simulink model "SigSourceBaseSignal"  (R2022b)
settings: Solver=VariableStepAuto  StartTime=0.0  StopTime=10.0  RelTol=1e-3
undefined symbols (not defined in the file): CarrierTs, CodeTs, gcbh, mdel, ModelInitial, rcfiltgaincompat, rsgenpoly, SignalSourceTs
libraries: commsynccomp2 x3, commblkintrlv2 x2, dspobslib x1, commblkcod2 x1, commfilt2 x1, commrandsrc3 x1, commdigbbndam3 x1, simulink x1, commdigbbndfm2 x1, commseqgen3 x1
settings Model: Creator=79327  LastModifiedBy=79327

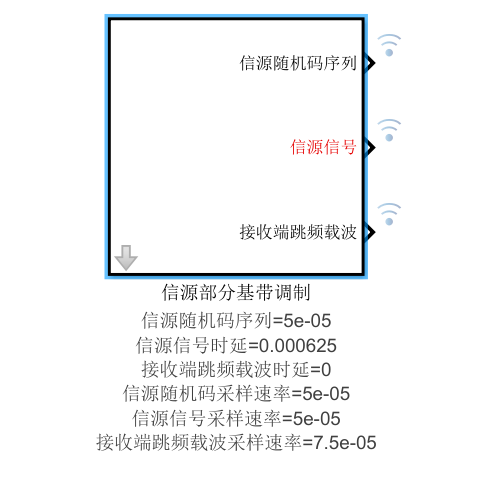
[thumbnail: Simulink's stored preview of the top-level diagram]
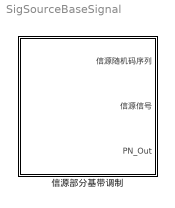
== system SigSourceBaseSignal ==
  信源部分基带调制 : Subsystem  InitFcn=ModelInitial(mdel,'信源部分基带调制',CodeTs,CarrierTs,SignalSourceTs)  TreatAsAtomicUnit=on  mask{SignalSource_Ts=SignalSourceTs, SampleFrame=3, M=15, PN_Generate=[1 0 0 0  0 1 1], PN_Init=[1 0 1 1 0 1], M_Freq=16, HopFrequencyStep=1e6, N=1500, Delay_HopFreq=0, Delay_SourceRand=5e-05, Delay_SignalSource=0.000625, CodeTs=CodeTs, CarrierTs=CarrierTs, SignalSourceTs=SignalSourceTs, T_HopFreq=7.5e-05, T_SourceRand=5e-05, T_SignalSource=5e-05}
      mask prompts: SignalSource_Ts "信源采样时间"; SampleFrame "信源随机码每帧的采样数"; M "信源M进制"; PN_Generate "PN生成器序列"; PN_Init "PN初始状态"; M_Freq "跳频的M进制"; HopFrequencyStep "跳频间隔"; N "输出跳频载波信号的维度"; Delay_HopFreq "接收端跳频载波的时延"; Delay_SourceRand "信源随机码的时延"; Delay_SignalSource "信源信号的时延"; CodeTs "采样时间"; CarrierTs "载波采样时间"; SignalSourceTs "信源采样时间"; T_HopFreq "接收端跳频载波的采样速率"; T_SourceRand "信源随机码的采样速率"; T_SignalSource "信源信号的采样速率"
      mask init:
      | %获得模块的句柄
      |              modelpath = gcb;
      |              model = getSimulinkBlockHandle(modelpath,true);
      |              buffer = getSimulinkBlockHandle([modelpath,'/Buffer3'],true);
      |              filter = getSimulinkBlockHandle([modelpath,'/Raised Cosine Transmit Filter1'],true);
      |             
      |              %计算buffer产生的时延
      |              buffer_outputsize = str2double(get_param(buffer,'N'));
      |              M = str2double(get_param(model,'M'));
      |              buffer_SPF = str2double(get_param(model,'SampleFrame'));
      |              BufferDelay = buffer_outputsize * SignalSourceTs * buffer_SPF / M;
      |             
      |              %计算filter产生的时延
      |              filter_span = str2double(get_param(filter,'filtSpan'));
      |              filterDelay = filter_span * SignalSourceTs * buffer_SPF / M / 2;
      |              
      |              %设置输出跳频载波信号的维度
      |              set_param(model,'N',num2str(round(SignalSourceTs * buffer_SPF / CarrierTs)));
      |              %设置滚降滤波的N
      |              set_param(filter,'N',num2str(round(SignalSourceTs * buffer_SPF / M / CarrierTs)));
      |     
      |              %设置信源随机码的时延
      |              set_param(model,'Delay_SourceRand',num2str(2 * SignalSourceTs));
      |              %设置信源信号的时延
      |              set_param(model,'Delay_SignalSource',num2str(BufferDelay + filterDelay));
      |              %设置接收端跳频载波的时延
      |              set_param(model,'Delay_HopFreq',num2str(0));
      |              %设置信源随机码的采样时间
      |              set_param(model,'T_SourceRand',num2str(CodeTs));
      |              %设置信源信号的采样时间
      |              set_param(model,'T_SignalSource',num2str(CodeTs));
      |              %设置接收端跳频载波的采样时间
      |              set_param(model,'T_HopFreq',num2str(buffer_SPF * SignalSourceTs));
      settings: AttributesFormatString=|
      | 信源随机码序列=%<Delay_SourceRand>
      | 信源信号时延=%<Delay_SignalSource>
      | 接收端跳频载波时延=%<Delay_HopFreq>
      | 信源随机码采样速率=%<T_SourceRand>
      | 信源信号采样速率=%<T_SignalSource>
      | 接收端跳频载波采样速率=%<T_HopFreq>
      mask DialogControl ParameterGroupVar Prompt: 参数
      mask DialogControl Container5 Prompt: 跳频参数
      mask DialogControl Container3 Prompt: 输出端的时延
      mask DialogControl Container4 Prompt: 输出端的采样速率
      mask DialogControl Container6 Prompt: 系统参数

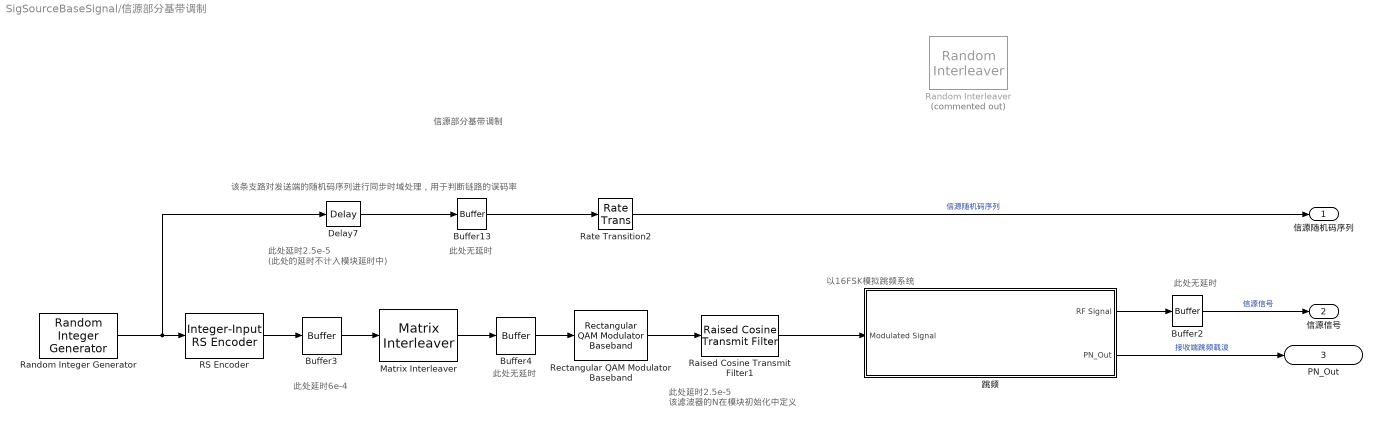
== system SigSourceBaseSignal/信源部分基带调制 ==
  note: 信源部分基带调制
  note: 此处延时2.5e-5
      | 该滤波器的N在模块初始化中定义
  note: 此处延时6e-4
  note: 此处无延时
  note: 该条支路对发送端的随机码序列进行同步时域处理，用于判断链路的误码率
  note: 此处延时2.5e-5
      | (此处的延时不计入模块延时中)
  note: 此处无延时
  note: 以16FSK模拟跳频系统
  note: 此处无延时
  Buffer13 : Buffer  N=1  OutputFrames=off
  Buffer2 : Buffer  N=1  OutputFrames=off
  Buffer3 : Buffer  N=120  OutputFrames=off
  Buffer4 : Buffer  N=M  OutputFrames=off
  Delay7 : dspobslib/Delay  InputProcessing=Columns as channels (frame based)  dly_unit=Samples  delay=1  ic_detail=off  dif_ic_for_ch=on  dif_ic_for_dly=off  ic=0  reset_popup=None
  Matrix Interleaver : commblkintrlv2/Matrix Interleaver  StatePerturbationForJacobian=1.0e-05  Nrows=12  Ncols=10
  RS Encoder : commblkcod2/Integer-Input RS Encoder  n=M  k=SampleFrame  specShortening=off  shortenedK=3  specGenPoly=off  genPoly=rsgenpoly(7,3)  specPrimPoly=off  prPoly=[1 0 1 1]  specPuncture=off  punctVec=[ones(2,1); zeros(2,1)]
  Raised Cosine Transmit Filter1 : commfilt2/Raised Cosine Transmit Filter  filtType=Square root  R=0.25  filtSpan=10  N=100  filterGain=rcfiltgaincompat(gcbh)  InputProcessing=Columns as channels (frame based)  RateOptions=Enforce single-rate processing  framing=Mute  checkCoeff=off  variableName=rcTxFilt1  checkGain=Normalized  sampMode=Mute  saveAsFlag=0  currentFiltSpan=10  D=(10)/2  launchFVT=on  roundingMode=Floor  overflowMode=off  coeffDataTypeStr=Inherit: Same word length as input  coeffMin=[]  coeffMax=[]  coeffLastDataTypeStr=Inherit: Same word length as input  outputDataTypeStr=Inherit: Same as accumulator  outputMin=[]  outputMax=[]  outputLastDataTypeStr=Inherit: Same as accumulator
  Random Interleaver : commblkintrlv2/Random Interleaver  Commented=on  StatePerturbationForJacobian=1.0e-05  N=120  seed=12345
  Random Integer Generator : commrandsrc3/Random Integer Generator  SetSize=M  SeedSource=Auto  Seed=4  SampleTime=SignalSourceTs  SamplesPerFrame=SampleFrame  OutputDataType=double  SimulateUsing=Interpreted execution
  Rate Transition2 : RateTransition  OutPortSampleTime=CarrierTs
  Rectangular QAM Modulator Baseband : commdigbbndam3/Rectangular QAM Modulator Baseband  M=16  InType=Integer  Enc=Gray  Mapping=[0:15]  PowType=Min. distance between symbols  MinDist=2  AvgPow=1  PeakPow=1  Ph=0  outDtype=double  outWordLen=16  outUDDataType=sfix(16)  outFracLenMode=Best precision  outFracLen=15  outDataTypeStr=double  outLastDataTypeStr=double
      settings: LibrarySourceBlock=|
      | commhdldigbbndam/Rectangular QAM
      | Modulator
      | Baseband
  跳频 : Subsystem  mask{PN_Generator=PN_Generate, PN_initial=PN_Init, M=M_Freq, FreqSeparation=HopFrequencyStep, T_input=SignalSourceTs * SampleFrame, T_min=CarrierTs}
      mask prompts: PN_Generator "PN序列的生成器系数"; PN_initial "PN序列的初始状态"; M "M进制跳频数(必须是2的倍数)"; FreqSeparation "跳频间隔"; T_input "输入信号的采样时间"; T_min "最小采样间隔"
      settings: AttributesFormatString=|
      | 输出信号的采样时间=%<T_input>
      | 一帧中最小采样单位时间是=%<T_min>
      mask DialogControl Container3 Prompt: PN序列参数
      mask DialogControl ParameterGroupVar Prompt: 跳频参数
  信源随机码序列 : Outport
  信源信号 : Outport  Port=2
  PN_Out : Outport  Port=3
  wires:
  Rectangular QAM Modulator Baseband/1 -> Raised Cosine Transmit Filter1/1
  RS Encoder/1 -> Buffer3/1
  Buffer4/1 -> Rectangular QAM Modulator Baseband/1
  Buffer3/1 -> Matrix Interleaver/1
  Matrix Interleaver/1 -> Buffer4/1
  Delay7/1 -> Buffer13/1
  Buffer13/1 -> Rate Transition2/1
  Rate Transition2/1 -> 信源随机码序列/1  "信源随机码序列"
  Random Integer Generator/1 -> Delay7/1, RS Encoder/1
  跳频/2(PN_Out) -> PN_Out/1  "接收端跳频载波"
  Buffer2/1 -> 信源信号/1  "信源信号"
  Raised Cosine Transmit Filter1/1 -> 跳频/1(Modulated Signal)
  跳频/1(RF Signal) -> Buffer2/1

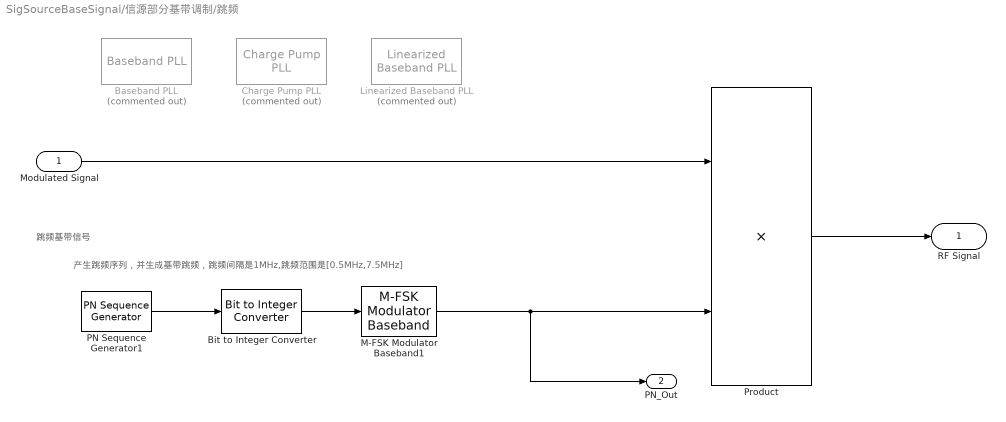
== system SigSourceBaseSignal/信源部分基带调制/跳频 ==
  note: 产生跳频序列，并生成基带跳频，跳频间隔是1MHz,跳频范围是[0.5MHz,7.5MHz]
  note: 跳频基带信号
  Modulated Signal : Inport
  Baseband PLL : commsynccomp2/Baseband PLL  Commented=on  Fn="[3.0002  0  40002]"  Fd="[1   67.46   2270.9   40002]"  Kvco=1
  Bit to Integer Converter : simulink/Logic and Bit Operations/Bit to Integer Converter  nbits=log2(M)  bitOrder=MSB first  signedOutputValues=Unsigned  outDtype=double  outDtypeSigned=Inherit via internal rule
  Charge Pump PLL : commsynccomp2/Charge Pump PLL  Commented=on  Fn="[3.0002  0  40002]"  Fd="[1   67.46   2270.9   40002]"  Kvco=1  Fc=100  Ph=0  Ac=1
  Linearized Baseband PLL : commsynccomp2/Linearized Baseband PLL  Commented=on  Fn="[3.0002  0  40002]"  Fd="[1   67.46   2270.9   40002]"  Kvco=1
  M-FSK Modulator Baseband1 : commdigbbndfm2/M-FSK Modulator Baseband  M=M  InType=Integer  Enc=Gray  freqSep=FreqSeparation  phaseType=Continuous  numSamp=(T_input / T_min)  RateOptions=Enforce single-rate processing  outDataType=double
  PN Sequence Generator1 : commseqgen3/PN Sequence Generator  poly=PN_Generator  ini_sta=PN_initial  outBitMaskSource=Dialog parameter  shift=0  outVarSiz=off  maxOutSizeMode=Dialog parameter  maxOutSize=[10 1]  Ts=(T_input / log2(M))  sampPerFrame=log2(M)  reset=off  bitPackedOutputs=off  outDataType=double  numPackedBits=5  bitPackDataSigned=off  bitPackedOutDType=double
  Product : Product
  RF Signal : Outport
  PN_Out : Outport  Port=2
  wires:
  Bit to Integer Converter/1 -> M-FSK Modulator Baseband1/1
  PN Sequence Generator1/1 -> Bit to Integer Converter/1
  Modulated Signal/1 -> Product/1
  Product/1 -> RF Signal/1
  M-FSK Modulator Baseband1/1 -> PN_Out/1, Product/2
